simulink model "Demo"  (R2017b)
settings: Solver=FixedStepDiscrete  StartTime=0.0  StopTime=inf  RelTol=1e-3  EnableMultiTasking=on
undefined symbols (not defined in the file or in its folder): none, videoinput
libraries: visionstatistics x2, imaqlib x1, visionsinks x1
settings Model: SimulationMode=accelerator  Creator=valakshe  LastModifiedBy=Vishwas Salunkhe
settings SolverCC: PositivePriorityOrder=on
settings OptimizationCC: DefaultParameterBehavior=Inlined  UseDivisionForNetSlopeComputation=on  UseFloatMulNetSlope=on  UseSpecifiedMinMax=on  InlineInvariantSignals=on  EnhancedBackFolding=on  BooleansAsBitfields=on  PassReuseOutputArgsAs=Individual arguments  ZeroExternalMemoryAtStartup=off  ZeroInternalMemoryAtStartup=off  NoFixptDivByZeroProtection=on  LifeSpan=inf  MaxStackSize=64  OptimizeBlockOrder=speed  DifferentSizesBufferReuse=on
settings DebuggingCC: SignalInfNanChecking=error  ReadBeforeWriteMsg=EnableAllAsError  WriteAfterWriteMsg=EnableAllAsError  WriteAfterReadMsg=EnableAllAsError  IntegerOverflowMsg=error  ParameterUnderflowMsg=error  ParameterPrecisionLossMsg=error  ParameterTunabilityLossMsg=error  UniqueDataStoreMsg=error  AssertControl=DisableAll  NonBusSignalsTreatedAsBus=error  SFInvalidInputDataAccessInChartInitDiag=error  SFTransitionOutsideNaturalParentDiag=error  SFUnreachableExecutionPathDiag=error  SFUndirectedBroadcastEventsDiag=error  IntegerSaturationMsg=error
settings HardwareCC: ProdBitPerPointer=32  ProdBitPerSizeT=32  ProdBitPerPtrDiffT=32  ProdLargestAtomicInteger=Long  ProdLargestAtomicFloat=Double  ProdWordSize=32  ProdLongLongMode=on  ProdHWDeviceType=ARM Compatible->ARM Cortex
settings SFSimCC: MATLABDynamicMemAlloc=off
settings RTWCC: SystemTargetFile=ert.tlc  HardwareBoard=Raspberry Pi  GenCodeOnly=on  PackageName=m.zip  TemplateMakefile=ert_default_tmf  GenerateReport=on  Toolchain=GNU GCC Raspberry Pi  BuildConfiguration=Faster Runs  IncludeHyperlinkInReport=on  LaunchReport=on  TargetLang=C++  GenerateTraceInfo=on  GenerateTraceReport=on  GenerateTraceReportSl=on  GenerateTraceReportSf=on  GenerateTraceReportEml=on  CheckMdlBeforeBuild=Warning
settings CodeAppCC: ForceParamTrailComments=on  IgnoreCustomStorageClasses=off  OperatorAnnotations=on  SimulinkDataObjDesc=on  SFDataObjDesc=on  MATLABFcnDesc=on  InsertBlockDesc=on  StateflowObjectComments=on  MATLABSourceComments=on  EnableCustomComments=on  ReqsInCode=on
settings ERTTargetCC: UtilityFuncGeneration=Shared location  CombineSignalStateStructs=on  SuppressErrorStatus=on  MultiInstanceERTCode=on  CodeInterfacePackaging=C++ class  SupportNonFinite=off  SupportVariableSizeSignals=on  ParenthesesLevel=Maximum  CastingMode=Standards  RootIOFormat=Structure reference  EnableSignedLeftShifts=off  EnableSignedRightShifts=off

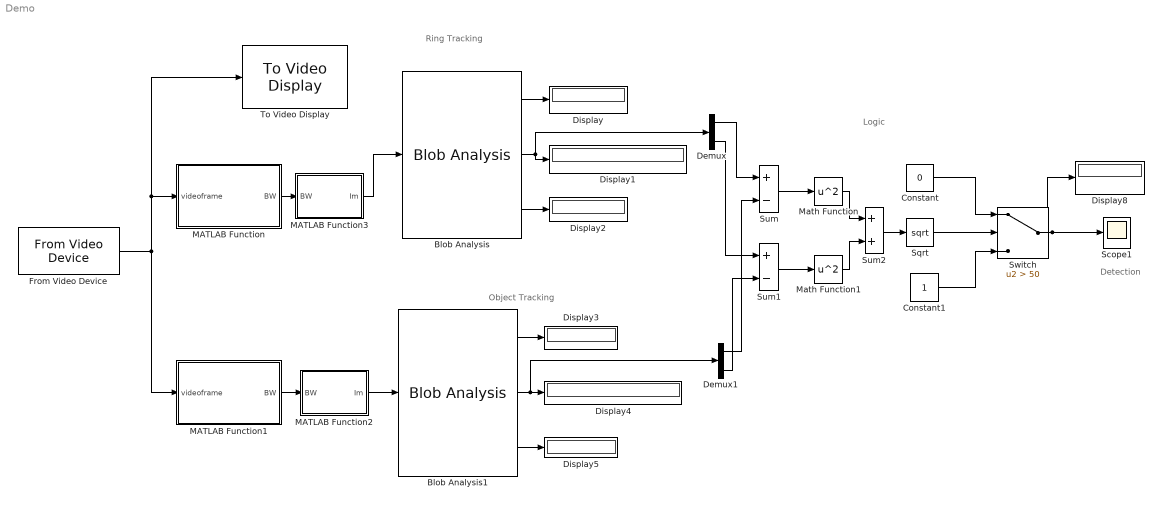
== system Demo ==
  note: Detection
  note: Logic
  note: Object Tracking
  note: Ring Tracking
  Blob Analysis : visionstatistics/Blob Analysis  Tag=vipblks_row_conv  area=on  centroid=on  bBox=off  majorAxis=off  minorAxis=off  angle=off  eccentricity=off  equivDiameterSq=off  extent=off  perimeter=off  maxBlobs=1  warnIfNumBlobsExceeded=on  isCount=on  useMinArea=on  minArea=2000  useMaxArea=on  maxArea=50000  excludeBorderBlob=off  outDT=double  isOutVarDim=off  isFill=on  fillValues=-1  conn=4  isLabel=off  outputMode=Binary point scaling  outputWordLength=32  outputFracLength=16  firstCoeffMode=Binary point scaling  firstCoeffWordLength=16  firstCoeffFracLength=14  secondCoeffMode=Binary point scaling  secondCoeffWordLength=32  secondCoeffFracLength=16  accumMode=Binary point scaling  accumWordLength=32  accumFracLength=0  prodOutputMode=Binary point scaling  prodOutputWordLength=32  prodOutputFracLength=16  roundingMode=Floor  overflowMode=off
      settings: SourceProductName=Computer Vision System Toolbox
  Blob Analysis1 : visionstatistics/Blob Analysis  Tag=vipblks_row_conv  area=on  centroid=on  bBox=off  majorAxis=off  minorAxis=off  angle=off  eccentricity=off  equivDiameterSq=off  extent=off  perimeter=off  maxBlobs=1  warnIfNumBlobsExceeded=on  isCount=on  useMinArea=on  minArea=2000  useMaxArea=on  maxArea=50000  excludeBorderBlob=off  outDT=double  isOutVarDim=off  isFill=on  fillValues=-1  conn=4  isLabel=off  outputMode=Binary point scaling  outputWordLength=32  outputFracLength=16  firstCoeffMode=Binary point scaling  firstCoeffWordLength=16  firstCoeffFracLength=14  secondCoeffMode=Binary point scaling  secondCoeffWordLength=32  secondCoeffFracLength=16  accumMode=Binary point scaling  accumWordLength=32  accumFracLength=0  prodOutputMode=Binary point scaling  prodOutputWordLength=32  prodOutputFracLength=16  roundingMode=Floor  overflowMode=off
      settings: SourceProductName=Computer Vision System Toolbox
  Constant : Constant  Value=0
  Constant1 : Constant
  Demux : Demux  Outputs=2
  Demux1 : Demux  Outputs=2
  Display{,1..5,8} (7 alike) : Display
  From Video Device : imaqlib/From Video Device  DeviceMenu=winvideo 1 (HP Truevision HD)  Device=winvideo 1 (HP Truevision HD)  ObjConstructor=videoinput('winvideo', 1)  VideoFormatMenu=MJPG_1280x720  VideoFormat=MJPG_1280x720  VideoSource=input1  ROIPosition=[0 0 720 1280]  EnableHWTrigger=off  TriggerConfiguration=none/none  SampleTime=1/30  OutputPortsMode=One multidimensional signal  DataType=single  CanDoHWTrigger=no  ReturnedColorSpace=grayscale  BlockHandle=25.0001  ROIWidth=1280  ROIHeight=720  ROIColumn=0  ROIRow=0  EngXMLPath=E:\MATLAB\R2017b\toolbox\imaq\imaq\private  DevXMLPath=C:\ProgramData\MATLAB\SupportPackages\R2017b\toolbox\imaq\supportpackages\genericvideo\adaptor\win64  EngLibPath=E:\MATLAB\R2017b\toolbox\imaq\imaqblks\imaqmex\win64  ColorSpace=grayscale  BayerSensorAlignment=grbg
      settings: SourceProductName=Image Acquisition Toolbox
  MATLAB Function : MATLAB Function  TreatAsAtomicUnit=on
  MATLAB Function1 : MATLAB Function  TreatAsAtomicUnit=on
  MATLAB Function2 : MATLAB Function  TreatAsAtomicUnit=on
  MATLAB Function3 : MATLAB Function  TreatAsAtomicUnit=on
  Math Function : Math  Operator=square  SaturateOnIntegerOverflow=on
  Math Function1 : Math  Operator=square  SaturateOnIntegerOverflow=on
  Scope1 : Scope
  Sqrt : Sqrt  SaturateOnIntegerOverflow=on
  Sum : Sum  Inputs=+-
  Sum1 : Sum  Inputs=+-
  Sum2 : Sum
  Switch : Switch  Criteria=u2 > Threshold  Threshold=50  OutMin=[50]  OutMax=[100]  RndMeth=Round  InputSameDT=on
  To Video Display : visionsinks/To Video Display  windowSizeMode=Normal  openAtMdlStart=on  fullScreen=off  videoWindowX=94  videoWindowY=166  saveWindowSize=off  videoWindowWidth=640  videoWindowHeight=480  inputColorFormat=RGB  inputType=Obsolete  imagePorts=One multidimensional signal  OutputDevice=On-screen video monitor  dataOrg=Column-major  isWindowOpen=off
      settings: SourceProductName=Computer Vision System Toolbox
  wires:
  Constant/1 -> Switch/1
  Switch/1 -> Display8/1, Scope1/1
  Math Function1/1 -> Sum2/2
  Constant1/1 -> Switch/3
  Sum2/1 -> Sqrt/1
  Blob Analysis1/1 -> Display3/1
  Sqrt/1 -> Switch/2
  Math Function/1 -> Sum2/1
  Demux1/2 -> Sum1/2
  Sum/1 -> Math Function/1
  Blob Analysis/1 -> Display/1
  Demux1/1 -> Sum/2
  Demux/2 -> Sum1/1
  Demux/1 -> Sum/1
  Blob Analysis1/3 -> Display5/1
  Blob Analysis1/2 -> Demux1/1, Display4/1
  MATLAB Function1/1(BW) -> MATLAB Function2/1(BW)
  Sum1/1 -> Math Function1/1
  Blob Analysis/2 -> Demux/1, Display1/1
  Blob Analysis/3 -> Display2/1
  MATLAB Function/1(BW) -> MATLAB Function3/1(BW)
  From Video Device/1 -> MATLAB Function/1(videoframe), To Video Display/1, MATLAB Function1/1(videoframe)
  MATLAB Function3/1(Im) -> Blob Analysis/1
  MATLAB Function2/1(Im) -> Blob Analysis1/1

== matlab function Demo/MATLAB Function1 ==
  data: videoframe input; BW output
function BW = fcn(videoframe)

    I = rgb2hsv(videoframe);

% Define thresholds for channel 1 based on histogram settings
    channel1Min = 0.476;
    channel1Max = 0.535;
    
    % Define thresholds for channel 2 based on histogram settings
    channel2Min = 0.486;
    channel2Max = 1.000;
    
    % Define thresholds for channel 3 based on histogram settings
    channel3Min = 0.257;
    channel3Max = 1.000;
    
    % Create mask based on chosen histogram thresholds
    BW = (I(:,:,1) >= channel1Min ) & (I(:,:,1) <= channel1Max) & ...
        (I(:,:,2) >= channel2Min ) & (I(:,:,2) <= channel2Max) & ...
        (I(:,:,3) >= channel3Min ) & (I(:,:,3) <= channel3Max);

== matlab function Demo/MATLAB Function ==
  data: videoframe input; BW output
function BW = fcn(videoframe)

    I = rgb2hsv(videoframe);

    % Define thresholds for channel 1 based on histogram settings
    channel1Min = 0.925;
    channel1Max = 0.032;
    
    % Define thresholds for channel 2 based on histogram settings
    channel2Min = 0.127;
    channel2Max = 1.000;
    
    % Define thresholds for channel 3 based on histogram settings
    channel3Min = 0.349;
    channel3Max = 1.000;
    
    % Create mask based on chosen histogram thresholds
    BW = ( (I(:,:,1) >= channel1Min) | (I(:,:,1) <= channel1Max) ) & ...
        (I(:,:,2) >= channel2Min ) & (I(:,:,2) <= channel2Max) & ...
        (I(:,:,3) >= channel3Min ) & (I(:,:,3) <= channel3Max);

== matlab function Demo/MATLAB Function2 ==
  data: BW input; Im output
function Im = fcn(BW)

 diskElem = strel('disk',3);
 Im = imopen(BW,diskElem);

== matlab function Demo/MATLAB Function3 ==
  data: BW input; Im output
function Im = fcn(BW)

 diskElem = strel('disk',3);
 Im = imopen(BW,diskElem);
